simulink model "xsg_multiply_add"  (R2015a)
settings: Solver=ode45  StartTime=0.0  StopTime=10.0  RelTol=1e-3
libraries: xbsIndex_r4 x58, s2ss x1
settings Model: Creator=ACS  LastModifiedBy=ACS

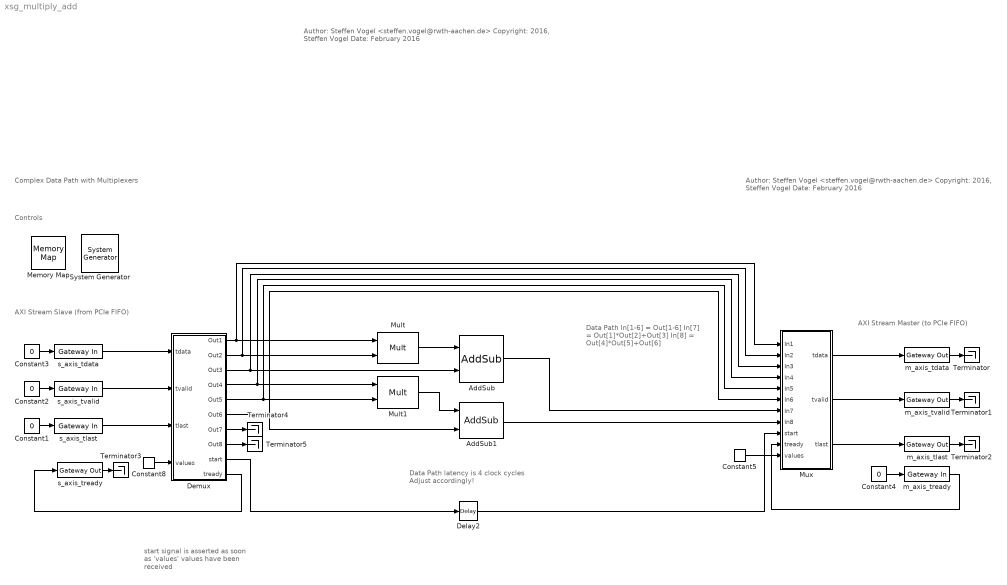
== system xsg_multiply_add ==
  note: start signal is asserted
      | as soon as  'values'
      | values have been received
  note: Data Path latency is 4 clock cycles
      | Adjust accordingly!
  note: Data Path
      |
      | In[1-6] = Out[1-6]
      | In[7] = Out[1]*Out[2]+Out[3]
      | In[8] = Out[4]*Out[5]+Out[6]
  note: AXI Stream Master
      | (to PCIe FIFO)
  note: AXI Stream Slave
      | (from PCIe FIFO)
  note: Controls
  note: Complex Data Path with Multiplexers
  note: Author: Steffen Vogel <steffen.vogel@rwth-aachen.de>
      | Copyright: 2016, Steffen Vogel
      | Date: February 2016
  note: Author: Steffen Vogel <steffen.vogel@rwth-aachen.de>
      | Copyright: 2016, Steffen Vogel
      | Date: February 2016
  " System Generator" : xbsIndex_r4/ System Generator  Tag=genX  xilinxfamily=virtex7  part=xc7vx485t  speed=-2  package=ffg1761  synthesis_tool=Vivado  clock_wrapper=Clock Enables  directory=D:/svo/gtfpga/sysgen/compiled/xsg_multiply_add  proj_type=Vivado  Synth_file=Vivado Synthesis Defaults  Impl_file=Vivado Implementation Defaults  testbench=off  simulink_period=1  sysclk_period=8  dcm_input_clock_period=10  incr_netlist=off  trim_vbits=Everywhere in SubSystem  dbl_ovrd=According to Block Masks  core_generation=According to Block Masks  run_coregen=off  deprecated_control=off  eval_field=0  block_type=sysgen
  AddSub : xbsIndex_r4/AddSub  mode=Addition  use_carryin=off  use_carryout=off  en=off  latency=1  precision=Full  arith_type=Unsigned  n_bits=16  bin_pt=14  quantization=Truncate  overflow=Wrap  use_behavioral_HDL=off  hw_selection=Fabric  pipelined=off  dbl_ovrd=off  block_type=addsub
  AddSub1 : xbsIndex_r4/AddSub  mode=Addition  use_carryin=off  use_carryout=off  en=off  latency=1  precision=Full  arith_type=Unsigned  n_bits=16  bin_pt=14  quantization=Truncate  overflow=Wrap  use_behavioral_HDL=off  hw_selection=Fabric  pipelined=off  dbl_ovrd=off  block_type=addsub
  Constant{1..4} (4 alike) : Constant  Value=0
  Constant5 : xbsIndex_r4/Constant  const=8  gui_display_data_type=Fixed-point  arith_type=Unsigned  n_bits=4  bin_pt=0  preci_type=Single  exp_width=8  frac_width=24  explicit_period=off  period=1  equ=P=C  opselect=C  inp2=PCIN>>17  opr=+  inp1=P  carry=CIN  dbl_ovrd=off  block_type=constant
  Constant8 : xbsIndex_r4/Constant  const=6  gui_display_data_type=Fixed-point  arith_type=Unsigned  n_bits=3  bin_pt=0  preci_type=Single  exp_width=8  frac_width=24  explicit_period=off  period=1  equ=P=C  opselect=C  inp2=PCIN>>17  opr=+  inp1=P  carry=CIN  dbl_ovrd=off  block_type=constant
  Delay2 : xbsIndex_r4/Delay  rst=off  infoeditControl=Selection of Reset will increase slice count due to use of real FFs and instead of SRLs  en=off  latency=4  reg_retiming=off  dbl_ovrd=off  block_type=delay
      settings: infoedit=Hardware notes: A delay line is a chain, each link of which is an SRL16 or SRL32 followed by a flip-flop.
  Demux : Subsystem
  Memory Map : s2ss/Memory Map  version=1.0  author=Steffen Vogel <stvogel@eonerc.rwth-aachen.de>  desc=FP Multiplication  company_url=http://www.acs.eonerc.rwth-aachen.de  vendor=acs.eonerc.rwth-aachen.de  vendor_display_name=Institute for Automation of Complex Power Systems, RWTH Aachen University  MaskMapDescription=test
  Mult : xbsIndex_r4/Mult  precision=Full  arith_type="Signed  (2's comp)"  n_bits=16  bin_pt=14  quantization=Truncate  overflow=Wrap  en=off  latency=3  use_behavioral_HDL=off  opt=Speed  use_embedded=on  optimum_pipeline=off  pipeline=on  dbl_ovrd=off  use_rpm=on  placement_style=Triangular  block_type=mult
  Mult1 : xbsIndex_r4/Mult  precision=Full  arith_type="Signed  (2's comp)"  n_bits=16  bin_pt=14  quantization=Truncate  overflow=Wrap  en=off  latency=3  use_behavioral_HDL=off  opt=Speed  use_embedded=on  optimum_pipeline=off  pipeline=on  dbl_ovrd=off  use_rpm=on  placement_style=Triangular  block_type=mult
  Mux : Subsystem
  Terminator{,1..5} (6 alike) : Terminator
  m_axis_tdata : xbsIndex_r4/Gateway Out  inherit_from_input=off  hdl_port=on  rows=1  columns=1  UseAsDAC=off  DACChannel='1'  interface=None  automatic_assignment=on  address_offset=hex2dec('00')  intf_name=''  intf_description=''  timing_constraint=None  locs_specified=off  LOCs={}  io_standard={}  block_type=gatewayout
  m_axis_tlast : xbsIndex_r4/Gateway Out  inherit_from_input=off  hdl_port=on  rows=1  columns=1  UseAsDAC=off  DACChannel='1'  interface=None  automatic_assignment=on  address_offset=hex2dec('00')  intf_name=''  intf_description=''  timing_constraint=None  locs_specified=off  LOCs={}  io_standard={}  block_type=gatewayout
  m_axis_tready : xbsIndex_r4/Gateway In  gui_display_data_type=Boolean  arith_type=Boolean  n_bits=16  bin_pt=14  preci_type=Single  exp_width=8  frac_width=24  rows=1  columns=1  quantization="Round  (unbiased: +/- Inf)"  overflow=Saturate  period=1  UseAsADC=off  ADCChannel='1'  interface=None  automatic_assignment=on  address_offset=hex2dec('00')  intf_name=''  intf_description=''  default_value=0  timing_constraint=None  locs_specified=off  LOCs={}  io_standard={}  inherit_from_input=off  hdl_port=on  dbl_ovrd=off  block_type=gatewayin
  m_axis_tvalid : xbsIndex_r4/Gateway Out  inherit_from_input=off  hdl_port=on  rows=1  columns=1  UseAsDAC=off  DACChannel='1'  interface=None  automatic_assignment=on  address_offset=hex2dec('00')  intf_name=''  intf_description=''  timing_constraint=None  locs_specified=off  LOCs={}  io_standard={}  block_type=gatewayout
  s_axis_tdata : xbsIndex_r4/Gateway In  gui_display_data_type=Floating-point  arith_type=Floating-point  n_bits=16  bin_pt=14  preci_type=Single  exp_width=8  frac_width=24  rows=1  columns=1  quantization="Round  (unbiased: +/- Inf)"  overflow=Saturate  period=1  UseAsADC=off  ADCChannel='1'  interface=None  automatic_assignment=on  address_offset=hex2dec('00')  intf_name=''  intf_description=''  default_value=0  timing_constraint=None  locs_specified=off  LOCs={}  io_standard={}  inherit_from_input=off  hdl_port=on  dbl_ovrd=off  block_type=gatewayin
  s_axis_tlast : xbsIndex_r4/Gateway In  gui_display_data_type=Boolean  arith_type=Boolean  n_bits=16  bin_pt=14  preci_type=Single  exp_width=8  frac_width=24  rows=1  columns=1  quantization="Round  (unbiased: +/- Inf)"  overflow=Saturate  period=1  UseAsADC=off  ADCChannel='1'  interface=None  automatic_assignment=on  address_offset=hex2dec('00')  intf_name=''  intf_description=''  default_value=0  timing_constraint=None  locs_specified=off  LOCs={}  io_standard={}  inherit_from_input=off  hdl_port=on  dbl_ovrd=off  block_type=gatewayin
  s_axis_tready : xbsIndex_r4/Gateway Out  inherit_from_input=off  hdl_port=on  rows=1  columns=1  UseAsDAC=off  DACChannel='1'  interface=None  automatic_assignment=on  address_offset=hex2dec('00')  intf_name=''  intf_description=''  timing_constraint=None  locs_specified=off  LOCs={}  io_standard={}  block_type=gatewayout
  s_axis_tvalid : xbsIndex_r4/Gateway In  gui_display_data_type=Boolean  arith_type=Boolean  n_bits=16  bin_pt=14  preci_type=Single  exp_width=8  frac_width=24  rows=1  columns=1  quantization="Round  (unbiased: +/- Inf)"  overflow=Saturate  period=1  UseAsADC=off  ADCChannel='1'  interface=None  automatic_assignment=on  address_offset=hex2dec('00')  intf_name=''  intf_description=''  default_value=0  timing_constraint=None  locs_specified=off  LOCs={}  io_standard={}  inherit_from_input=off  hdl_port=on  dbl_ovrd=off  block_type=gatewayin
  wires:
  s_axis_tvalid/1 -> Demux/2(tvalid)
  s_axis_tlast/1 -> Demux/3(tlast)
  m_axis_tdata/1 -> Terminator/1
  m_axis_tvalid/1 -> Terminator1/1
  m_axis_tlast/1 -> Terminator2/1
  Constant1/1 -> s_axis_tlast/1
  Constant2/1 -> s_axis_tvalid/1
  Constant3/1 -> s_axis_tdata/1
  Constant4/1 -> m_axis_tready/1
  s_axis_tready/1 -> Terminator3/1
  Mult/1 -> AddSub/1
  Mult1/1 -> AddSub1/1
  s_axis_tdata/1 -> Demux/1(tdata)
  Demux/1(Out1) -> Mux/1(In1), Mult/1
  Demux/2(Out2) -> Mux/2(In2), Mult/2
  Demux/3(Out3) -> Mux/3(In3), AddSub/2
  Demux/4(Out4) -> Mux/4(In4), Mult1/1
  Demux/5(Out5) -> Mult1/2, Mux/5(In5)
  Demux/6(Out6) -> AddSub1/2, Mux/6(In6)
  Mux/1(tdata) -> m_axis_tdata/1
  Mux/2(tvalid) -> m_axis_tvalid/1
  Mux/3(tlast) -> m_axis_tlast/1
  Demux/9(start) -> Delay2/1
  Delay2/1 -> Mux/9(start)
  AddSub/1 -> Mux/7(In7)
  AddSub1/1 -> Mux/8(In8)
  m_axis_tready/1 -> Mux/10(tready)
  Demux/7(Out7) -> Terminator4/1
  Demux/8(Out8) -> Terminator5/1
  Constant8/1 -> Demux/4(values)
  Demux/10(tready) -> s_axis_tready/1
  Constant5/1 -> Mux/11(values)

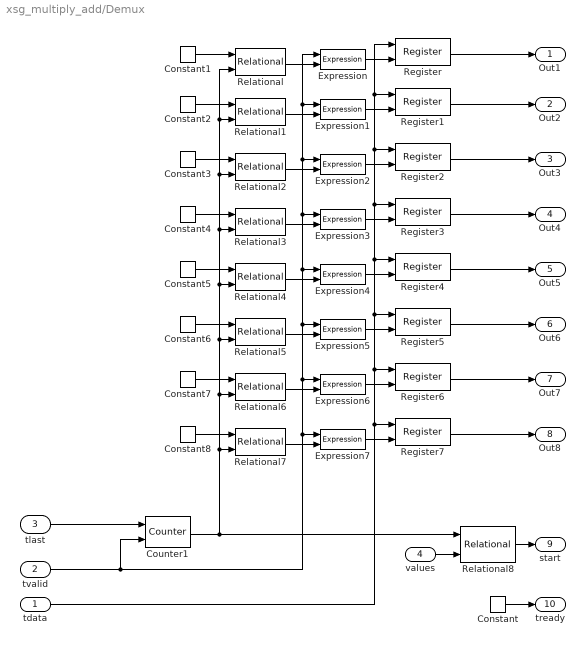
== system xsg_multiply_add/Demux ==
  tdata : Inport
  tvalid : Inport  Port=2
  tlast : Inport  Port=3
  values : Inport  Port=4
  Constant : xbsIndex_r4/Constant  const=1.0  gui_display_data_type=Boolean  arith_type=Boolean  n_bits=16  bin_pt=14  preci_type=Single  exp_width=8  frac_width=24  explicit_period=off  period=1  equ=P=C  opselect=C  inp2=PCIN>>17  opr=+  inp1=P  carry=CIN  dbl_ovrd=off  block_type=constant
  Constant{1..8} (8 alike) : xbsIndex_r4/Constant  const=0  gui_display_data_type=Fixed-point  arith_type=Unsigned  n_bits=3  bin_pt=0  preci_type=Single  exp_width=8  frac_width=24  explicit_period=off  period=1  equ=P=C  opselect=C  inp2=PCIN>>17  opr=+  inp1=P  carry=CIN  dbl_ovrd=off  block_type=constant
  Counter1 : xbsIndex_r4/Counter  cnt_type=Free Running  cnt_to=Inf  operation=Up  start_count=0  cnt_by_val=1  arith_type=Unsigned  n_bits=3  bin_pt=0  load_pin=off  rst=on  en=on  explicit_period=on  period=1  use_behavioral_HDL=off  implementation=Fabric  dbl_ovrd=off  block_type=counter
  Expression{,1..7} (8 alike) : xbsIndex_r4/Expression  expression=a & b  align_bp=on  en=off  latency=0  precision=Full  arith_type=Unsigned  n_bits=16  bin_pt=0  dbl_ovrd=off  block_type=expr
  Register{,1..7} (8 alike) : xbsIndex_r4/Register  init=0  rst=off  en=on  dbl_ovrd=off  block_type=register
  Relational{,1..7} (8 alike) : xbsIndex_r4/Relational  mode=a=b  op_type=Bool  en=off  latency=0  dbl_ovrd=off  block_type=relational
  Relational8 : xbsIndex_r4/Relational  mode=a=b  op_type=Bool  en=off  latency=1  dbl_ovrd=off  block_type=relational
  Out1 : Outport
  Out2 : Outport  Port=2
  Out3 : Outport  Port=3
  Out4 : Outport  Port=4
  Out5 : Outport  Port=5
  Out6 : Outport  Port=6
  Out7 : Outport  Port=7
  Out8 : Outport  Port=8
  start : Outport  Port=9
  tready : Outport  Port=10
  wires:
  Register1/1 -> Out2/1
  Register/1 -> Out1/1
  Expression3/1 -> Register3/2
  Expression2/1 -> Register2/2
  tdata/1 -> Register7/1, Register6/1, Register/1, Register1/1, Register2/1, Register3/1, Register4/1, Register5/1
  Expression1/1 -> Register1/2
  Counter1/1 -> Relational8/1, Relational7/2, Relational6/2, Relational5/2, Relational4/2, Relational3/2, Relational2/2, Relational1/2, Relational/2
  Expression/1 -> Register/2
  Relational/1 -> Expression/2
  Relational4/1 -> Expression4/2
  Register3/1 -> Out4/1
  Register4/1 -> Out5/1
  Expression4/1 -> Register4/2
  Register2/1 -> Out3/1
  Relational1/1 -> Expression1/2
  Register5/1 -> Out6/1
  Relational3/1 -> Expression3/2
  Relational2/1 -> Expression2/2
  tlast/1 -> Counter1/1
  Relational5/1 -> Expression5/2
  Expression5/1 -> Register5/2
  tvalid/1 -> Counter1/2, Expression7/1, Expression6/1, Expression/1, Expression1/1, Expression2/1, Expression3/1, Expression4/1, Expression5/1
  Relational8/1 -> start/1
  Relational6/1 -> Expression6/2
  Expression7/1 -> Register7/2
  Expression6/1 -> Register6/2
  Register6/1 -> Out7/1
  Register7/1 -> Out8/1
  Relational7/1 -> Expression7/2
  values/1 -> Relational8/2
  Constant/1 -> tready/1
  Constant2/1 -> Relational1/1
  Constant1/1 -> Relational/1
  Constant3/1 -> Relational2/1
  Constant4/1 -> Relational3/1
  Constant5/1 -> Relational4/1
  Constant6/1 -> Relational5/1
  Constant7/1 -> Relational6/1
  Constant8/1 -> Relational7/1

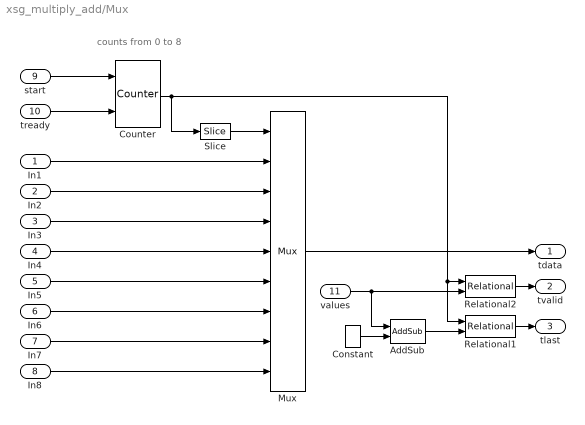
== system xsg_multiply_add/Mux ==
  note: counts from 0 to 8
  In1 : Inport
  In2 : Inport  Port=2
  In3 : Inport  Port=3
  In4 : Inport  Port=4
  In5 : Inport  Port=5
  In6 : Inport  Port=6
  In7 : Inport  Port=7
  In8 : Inport  Port=8
  start : Inport  Port=9
  tready : Inport  Port=10
  values : Inport  Port=11
  AddSub : xbsIndex_r4/AddSub  mode=Subtraction  use_carryin=off  use_carryout=off  en=off  latency=0  precision=Full  arith_type=Unsigned  n_bits=16  bin_pt=14  quantization=Truncate  overflow=Wrap  use_behavioral_HDL=off  hw_selection=Fabric  pipelined=off  dbl_ovrd=off  block_type=addsub
  Constant : xbsIndex_r4/Constant  const=1  gui_display_data_type=Fixed-point  arith_type=Signed (2's comp)  n_bits=4  bin_pt=0  preci_type=Single  exp_width=8  frac_width=24  explicit_period=off  period=1  equ=P=C  opselect=C  inp2=PCIN>>17  opr=+  inp1=P  carry=CIN  dbl_ovrd=off  block_type=constant
  Counter : xbsIndex_r4/Counter  cnt_type=Count Limited  cnt_to=8  operation=Up  start_count=0  cnt_by_val=1  arith_type=Unsigned  n_bits=4  bin_pt=0  load_pin=off  rst=on  en=on  explicit_period=on  period=1  use_behavioral_HDL=off  implementation=Fabric  dbl_ovrd=off  block_type=counter
  Mux : xbsIndex_r4/Mux  inputs=8  en=off  latency=0  precision=Full  arith_type=Unsigned  n_bits=16  bin_pt=14  quantization=Truncate  overflow=Wrap  dbl_ovrd=off  block_type=mux
  Relational1 : xbsIndex_r4/Relational  mode=a=b  op_type=Bool  en=off  latency=0  dbl_ovrd=off  block_type=relational
  Relational2 : xbsIndex_r4/Relational  mode=a<b  op_type=Bool  en=off  latency=0  dbl_ovrd=off  block_type=relational
  Slice : xbsIndex_r4/Slice  nbits=3  boolean_output=off  mode=Upper Bit Location + Width  bit1=0  base1=MSB of Input  bit0=0  base0=LSB of Input  dbl_ovrd=off  block_type=slice
  tdata : Outport
  tvalid : Outport  Port=2
  tlast : Outport  Port=3
  wires:
  In1/1 -> Mux/2
  In2/1 -> Mux/3
  Mux/1 -> tdata/1
  start/1 -> Counter/1
  In3/1 -> Mux/4
  In4/1 -> Mux/5
  In5/1 -> Mux/6
  In6/1 -> Mux/7
  In7/1 -> Mux/8
  In8/1 -> Mux/9
  tready/1 -> Counter/2
  Relational1/1 -> tlast/1
  Counter/1 -> Slice/1, Relational2/1, Relational1/1
  Slice/1 -> Mux/1
  Relational2/1 -> tvalid/1
  values/1 -> AddSub/1, Relational2/2
  AddSub/1 -> Relational1/2
  Constant/1 -> AddSub/2
